simulink model "question4"  (R2019b)
settings: Solver=VariableStepAuto  StartTime=0.0  StopTime=0.3  RelTol=1e-3
settings Model: Creator=theojanson  LastModifiedBy=theojanson

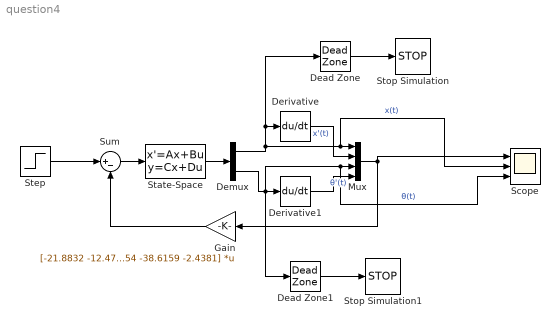
== system question4 ==
  Dead Zone : DeadZone  SaturateOnIntegerOverflow=on
  Dead Zone1 : DeadZone  LowerValue=-0.1  UpperValue=0.1  SaturateOnIntegerOverflow=on
  Demux : Demux  Outputs=2
  Derivative : Derivative
  Derivative1 : Derivative
  Gain : Gain  Gain=[-21.8832 -12.4754 -38.6159 -2.4381]  Multiplication=Matrix(K*u) (u vector)
  Mux : Mux
  Scope : Scope  NumInputPorts=3
  State-Space : StateSpace  A=[0 1 0 0 ; 0 -14.4899 -1.9749 0 ; 0 0 0 1 ; 0 86.2495 58.3333 0]  B=[0 ; 3.255 ; 0 ; -19.3751]  C=[1 0 0 0 ; 0 0 1 0]  D=[0;0]  InitialCondition=[0 0 0.09 1]
  Step : Step  SampleTime=0
  Stop Simulation : Stop
  Stop Simulation1 : Stop
  Sum : Sum  Inputs=|+-
  wires:
  State-Space/1 -> Demux/1
  Demux/1 -> Derivative/1, Dead Zone/1, Scope/2, Mux/1  "x(t)"
  Derivative/1 -> Mux/2  "x'(t)"
  Demux/2 -> Scope/3, Mux/3, Derivative1/1, Dead Zone1/1  "θ(t)"
  Derivative1/1 -> Mux/4  "θ'(t)"
  Mux/1 -> Scope/1, Gain/1
  Sum/1 -> State-Space/1
  Step/1 -> Sum/1
  Gain/1 -> Sum/2
  Dead Zone/1 -> Stop Simulation/1
  Dead Zone1/1 -> Stop Simulation1/1
